simulink library "FixedLib"  (R2022b)
settings: Solver=VariableStepAuto  StartTime=0.0  StopTime=10.0  RelTol=1e-3
undefined symbols (not defined in the file): T1Break, T1Data
settings Model: Creator=amyyang  LastModifiedBy=amyyang

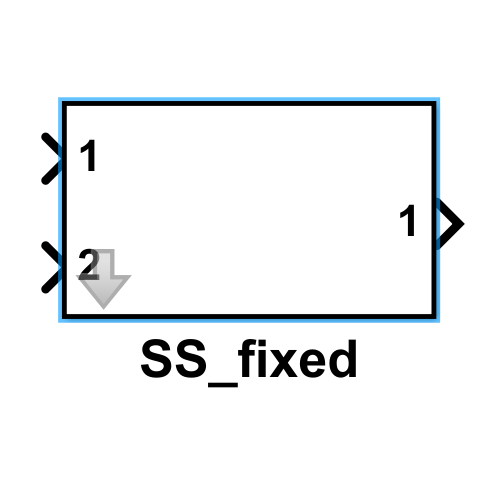
[thumbnail: Simulink's stored preview of the top-level diagram]
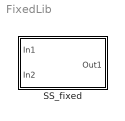
== system FixedLib ==
  SS_fixed : Subsystem  TreatAsAtomicUnit=on  RTWFcnName=myfun_Fixed  RTWFileName=myfile  mask(SSDemo){x=T1Break, y=T1Data}
      mask prompts: x "Break points (X data):"; y "Output values (Y data):"
      mask help: Example to show code reuse. This example has two parameters for a lookup table.
      settings: RTWFcnNameOpts=User specified

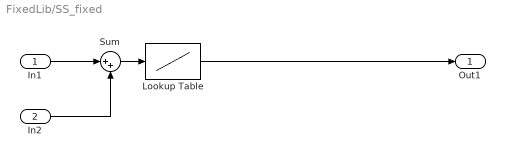
== system FixedLib/SS_fixed ==
  In1 : Inport
  In2 : Inport  Port=2
  Lookup Table : Lookup_n-D  NumberOfTableDimensions=1  BreakpointsForDimension1=x  Table=y
  Sum : Sum  Inputs=|++
  Out1 : Outport  VectorParamsAs1DForOutWhenUnconnected=off
  wires:
  Sum/1 -> Lookup Table/1
  In2/1 -> Sum/2
  In1/1 -> Sum/1
  Lookup Table/1 -> Out1/1
